simulink model "ADCS_r2017b"  (R2018a)
settings: Solver=FixedStepAuto  StartTime=0.0  StopTime=end_time  FixedStep=delta_t  RelTol=1e-3
undefined symbols (not defined in the file or in its folder): delta_t, SC, SS
libraries: sharedutil x5, vrlib x2
(part 1 of 3)
settings Model: Creator=azufall  LastModifiedBy=Hridu
settings DebuggingCC: AlgebraicLoopMsg=none

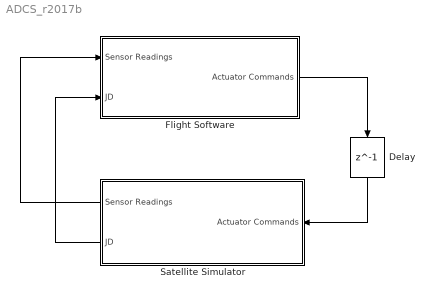
== system ADCS_r2017b ==
  Delay : Delay  DelayLength=1  InitialCondition=0
  Flight Software : Subsystem
  Satellite Simulator : Subsystem
  wires:
  Flight Software/1(Actuator Commands) -> Delay/1
  Satellite Simulator/2(JD) -> Flight Software/2(JD)
  Satellite Simulator/1(Sensor Readings) -> Flight Software/1(Sensor Readings)
  Delay/1 -> Satellite Simulator/1(Actuator Commands)

== system ADCS_r2017b/Flight Software ==
  Sensor Readings : Inport
  JD : Inport  Port=2
  Bus Selector : BusSelector  OutputSignals=gyro meas,sun meas,star meas
  Resolution Error : Rounding
  Subsystems : Subsystem
  Thrust command : Gain  Gain=SC.RCS.num_bits
  Thrust command1 : Gain  Gain=1/SC.RCS.num_bits
  Actuator Commands : Outport
  wires:
  Subsystems/1(RCS Command) -> Thrust command/1
  Sensor Readings/1 -> Bus Selector/1
  Bus Selector/1 -> Subsystems/1(Gyro)  "<gyro meas>"
  Bus Selector/3 -> Subsystems/3(Star Tracker)  "<star meas>"
  JD/1 -> Subsystems/4(JD)
  Thrust command/1 -> Resolution Error/1
  Resolution Error/1 -> Thrust command1/1
  Bus Selector/2 -> Subsystems/2(Sun Sensor)  "<sun meas>"
  Thrust command1/1 -> Actuator Commands/1

== system ADCS_r2017b/Satellite Simulator ==
  Actuator Commands : Inport
  Actuators : Subsystem
  Constant : Constant  Value=0
  Constant1 : Constant  Value=[0;0;0]
  Constant2 : Constant  Value=[0;0;0]
  Delay : Delay  DelayLength=1  InitialConditionSource=Input port  InitialCondition=0
      settings: InputPortMap=u0,p4
  Delay1 : Delay  DelayLength=1  InitialConditionSource=Input port  InitialCondition=0
      settings: InputPortMap=u0,p4
  Environment : Subsystem
  External Forces and Torques : Subsystem
  Kinematics : Subsystem
  Sensors : Subsystem
  Sum : Sum  Inputs=++|
  Sum1 : Sum  Inputs=++|
  Time Model : Subsystem
  Sensor Readings : Outport
  JD : Outport  Port=2  PortDimensions=1
  wires:
  Kinematics/3(Omega) -> Sensors/3(w_body2eci)
  Sensors/1(Sensor Readings) -> Sensor Readings/1
  Time Model/1(JD) -> External Forces and Torques/8(JD), Kinematics/3(JD), Environment/1(JD), JD/1
  Environment/1(sun_eci) -> Sensors/2(Sun info), External Forces and Torques/4(sun_eci)
  Environment/2(moon_eci) -> External Forces and Torques/5(moon_eci)
  Environment/3(Mag) -> External Forces and Torques/6(Mag)
  External Forces and Torques/1(a_eci) -> Sum/2
  External Forces and Torques/2(tor_body) -> Sum1/2
  Kinematics/2(v_eci) -> External Forces and Torques/2(Velocity)
  Kinematics/4(Coordinate Transforms) -> Environment/3(Coordinate Transforms), Sensors/4(Coordinate Transforms), Actuators/3(Coordinate Transforms), External Forces and Torques/3(Coordinate Transforms)
  Actuators/1(a_eci) -> Sum/1
  Actuators/2(torque_body) -> Sum1/1
  Kinematics/1(r_eci) -> Sensors/1(Position), Environment/2(r_eci), External Forces and Torques/1(Position)
  Environment/4(Eclipse) -> Sensors/6(eclipse), External Forces and Torques/7(Eclipse)
  Kinematics/5(q) -> Sensors/5(q_eci2body)
  Actuator Commands/1 -> Actuators/1(RCS Command)
  Constant/1 -> Actuators/2(Other Actuator?)
  Sum1/1 -> Delay/1
  Sum/1 -> Delay1/1
  Delay1/1 -> Kinematics/1(a_eci)
  Constant1/1 -> Delay1/2
  Constant2/1 -> Delay/2
  Delay/1 -> Kinematics/2(Torque_body)

== system ADCS_r2017b/Flight Software/Subsystems ==
  Gyro : Inport
  Sun Sensor : Inport  Port=2
  Star Tracker : Inport  Port=3
  JD : Inport  Port=4
  Mode Selection : Subsystem
  RCS Controller : Subsystem
  Sensor Processing : Subsystem
  To Workspace : ToWorkspace  VariableName=mode_out  SampleTime=-1
  RCS Command : Outport
  wires:
  Gyro/1 -> Sensor Processing/1(Gyro_raw)
  Sun Sensor/1 -> Sensor Processing/2(Sun_raw)
  Star Tracker/1 -> Sensor Processing/3(Star_raw)
  Sensor Processing/1(Gyro_filtered) -> RCS Controller/2(Gyro), Mode Selection/1(Gyro)
  Sensor Processing/4(Eclipse) -> RCS Controller/7(eclipse), Mode Selection/2(Eclipse)
  JD/1 -> RCS Controller/6(JD), Mode Selection/3(Time)
  RCS Controller/1(RCS_Command) -> RCS Command/1
  Mode Selection/2(S/C Mode) -> To Workspace/1, RCS Controller/1(Mode)
  Mode Selection/1(Controller Gains) -> RCS Controller/5(Gains)
  Sensor Processing/3(Star_filtered) -> RCS Controller/4(Star)
  Sensor Processing/2(Sun_filtered) -> RCS Controller/3(Sun)

== system ADCS_r2017b/Satellite Simulator/Actuators ==
  RCS Command : Inport
  Other Actuator? : Inport  Port=2
  Coordinate Transforms : Inport  Port=3
  Bus Selector : BusSelector  OutputSignals=R_eci2body
  Constant : Constant  Value=SC.RCS.moment_arms
  Constant1 : Constant  Value=SC.RCS.max_thrust
  Constant2 : Constant  Value=SC.RCS.dir
  Constant3 : Constant  Value=SC.RCS.noise
  Constant4 : Constant  Value=SC.RCS.bias
  Gain : Gain  Gain=1/SC.mass_properties.mass
  Math Function : Math  Operator=transpose  SaturateOnIntegerOverflow=on
  Matrix Multiply : Product  Multiplication=Matrix(*)
  RCS Model : MATLAB Function  TreatAsAtomicUnit=on
  Terminator : Terminator
  To Workspace : ToWorkspace  VariableName=act_tor_body  SampleTime=-1
  To Workspace1 : ToWorkspace  VariableName=RCS_cmds  SampleTime=-1
  a_eci : Outport
  torque_body : Outport  Port=2
  wires:
  RCS Command/1 -> To Workspace1/1, RCS Model/1(command)
  RCS Model/2(torque_body) -> To Workspace/1, torque_body/1
  Other Actuator?/1 -> Terminator/1
  Coordinate Transforms/1 -> Bus Selector/1
  Bus Selector/1 -> Math Function/1  "<R_eci2body>"
  RCS Model/1(force_body) -> Matrix Multiply/2
  Math Function/1 -> Matrix Multiply/1  "R_body2eci"
  Constant/1 -> RCS Model/2(moment_arm)
  Constant1/1 -> RCS Model/4(max_thrust)
  Constant2/1 -> RCS Model/3(norm_dir)
  Gain/1 -> a_eci/1
  Matrix Multiply/1 -> Gain/1
  Constant3/1 -> RCS Model/5(noise)
  Constant4/1 -> RCS Model/6(bias)

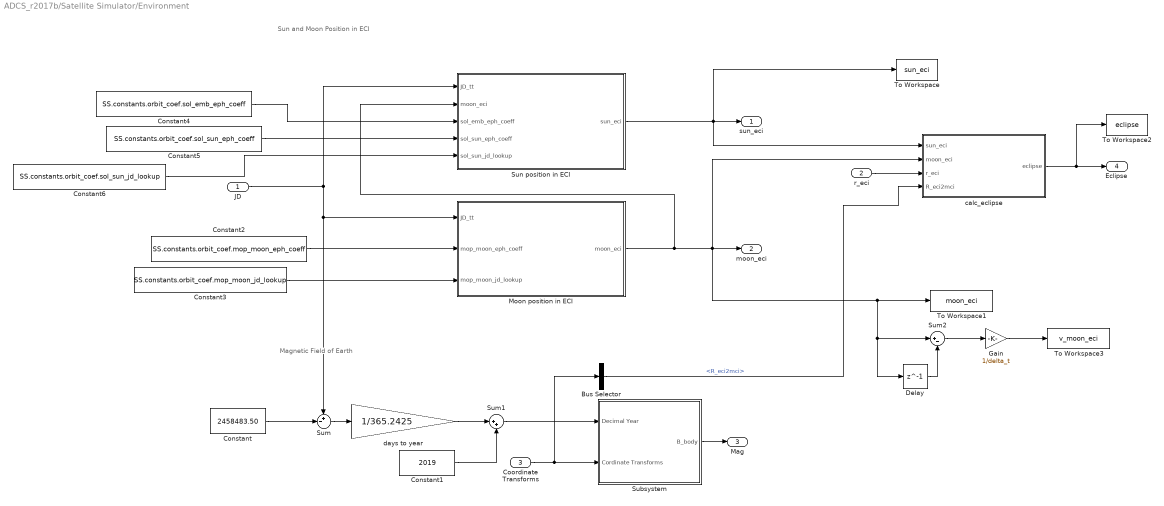
== system ADCS_r2017b/Satellite Simulator/Environment ==
  note: Sun and Moon Position in ECI
  note: Magnetic Field of Earth
  JD : Inport
  r_eci : Inport  Port=2
  Coordinate Transforms : Inport  Port=3
  Bus Selector : BusSelector  OutputSignals=R_eci2mci
  Constant : Constant  Value=2458483.50
  Constant1 : Constant  Value=2019
  Constant2 : Constant  Value=SS.constants.orbit_coef.mop_moon_eph_coeff
  Constant3 : Constant  Value=SS.constants.orbit_coef.mop_moon_jd_lookup
  Constant4 : Constant  Value=SS.constants.orbit_coef.sol_emb_eph_coeff
  Constant5 : Constant  Value=SS.constants.orbit_coef.sol_sun_eph_coeff
  Constant6 : Constant  Value=SS.constants.orbit_coef.sol_sun_jd_lookup
  Delay : Delay  DelayLength=1  InitialCondition=0
  Gain : Gain  Gain=1/delta_t
  Moon position in ECI : MATLAB Function  TreatAsAtomicUnit=on
  Subsystem : Subsystem
  Sum : Sum  Inputs=+-|
  Sum1 : Sum  Inputs=|++
  Sum2 : Sum  Inputs=|+-
  Sun position in ECI : MATLAB Function  TreatAsAtomicUnit=on
  To Workspace : ToWorkspace  VariableName=sun_eci  SampleTime=-1
  To Workspace1 : ToWorkspace  VariableName=moon_eci  SampleTime=-1
  To Workspace2 : ToWorkspace  VariableName=eclipse  SampleTime=-1
  To Workspace3 : ToWorkspace  VariableName=v_moon_eci  SampleTime=-1
  calc_eclipse : MATLAB Function  TreatAsAtomicUnit=on
  days to year : Gain  Gain=1/365.2425
  sun_eci : Outport
  moon_eci : Outport  Port=2
  Mag : Outport  Port=3
  Eclipse : Outport  Port=4
  wires:
  Moon position in ECI/1(moon_eci) -> Sun position in ECI/2(moon_eci), calc_eclipse/2(moon_eci), moon_eci/1, Delay/1, Sum2/1, To Workspace1/1
  Subsystem/1(B_body) -> Mag/1
  calc_eclipse/1(eclipse) -> To Workspace2/1, Eclipse/1
  JD/1 -> Sum/1, Moon position in ECI/1(JD_tt), Sun position in ECI/1(JD_tt)
  Sun position in ECI/1(sun_eci) -> sun_eci/1, To Workspace/1, calc_eclipse/1(sun_eci)
  r_eci/1 -> calc_eclipse/3(r_eci)
  Sum/1 -> days to year/1
  Constant/1 -> Sum/2
  days to year/1 -> Sum1/1
  Sum1/1 -> Subsystem/1(Decimal Year)
  Constant1/1 -> Sum1/2
  Coordinate Transforms/1 -> Bus Selector/1, Subsystem/2(Cordinate Transforms)
  Constant2/1 -> Moon position in ECI/2(mop_moon_eph_coeff)
  Constant3/1 -> Moon position in ECI/3(mop_moon_jd_lookup)
  Constant4/1 -> Sun position in ECI/3(sol_emb_eph_coeff)
  Constant5/1 -> Sun position in ECI/4(sol_sun_eph_coeff)
  Constant6/1 -> Sun position in ECI/5(sol_sun_jd_lookup)
  Bus Selector/1 -> calc_eclipse/4(R_eci2mci)  "<R_eci2mci>"
  Delay/1 -> Sum2/2
  Sum2/1 -> Gain/1
  Gain/1 -> To Workspace3/1

== system ADCS_r2017b/Satellite Simulator/External Forces and Torques ==
  Position : Inport
  Velocity : Inport  Port=2
  Coordinate Transforms : Inport  Port=3
  sun_eci : Inport  Port=4
  moon_eci : Inport  Port=5
  Mag : Inport  Port=6
  Eclipse : Inport  Port=7
  JD : Inport  Port=8
  External Forces : Subsystem
  External Torques : Subsystem
  a_eci : Outport
  tor_body : Outport  Port=2
  wires:
  Position/1 -> External Forces/1(r_eci), External Torques/3(r_eci)
  moon_eci/1 -> External Forces/5(moon eci)
  sun_eci/1 -> External Forces/4(Sun eci)
  Velocity/1 -> External Forces/2(Velocity)
  Coordinate Transforms/1 -> External Torques/5(Coordinate Transforms), External Forces/3(Coordinate Transforms)
  External Forces/1(a_eci) -> a_eci/1
  External Torques/1(Torques) -> tor_body/1
  Eclipse/1 -> External Forces/6(Eclipse)
  Mag/1 -> External Torques/4(Mag)
  External Forces/2(Aero_body) -> External Torques/1(Force_aero_body)
  External Forces/3(SRP_body) -> External Torques/2(Force_SRP_body)
  JD/1 -> External Forces/7(JD)

== system ADCS_r2017b/Satellite Simulator/Kinematics ==
  a_eci : Inport
  Torque_body : Inport  Port=2
  JD : Inport  Port=3  PortDimensions=1
  Backup Rotation Kinematics : Subsystem
  Calc Coordinate Transforms : Subsystem
  Position Kinematics : Subsystem
  Rotation Kinematics : Subsystem
  To Workspace : ToWorkspace  VariableName=q_out  SampleTime=-1
  To Workspace1 : ToWorkspace  VariableName=omega_out  SampleTime=-1
  To Workspace2 : ToWorkspace  VariableName=e_out  SampleTime=-1
  To Workspace3 : ToWorkspace  VariableName=omega_euler_out  SampleTime=-1
  r_eci : Outport
  v_eci : Outport  Port=2
  Omega : Outport  Port=3
  Coordinate Transforms : Outport  Port=4
  q : Outport  Port=5
  wires:
  a_eci/1 -> Position Kinematics/1(a_eci)
  Torque_body/1 -> Backup Rotation Kinematics/1(torque_body), Rotation Kinematics/1(torque_body)
  Rotation Kinematics/2(w_body_eci) -> To Workspace1/1, Omega/1
  Calc Coordinate Transforms/1(Coordinate Transforms) -> Coordinate Transforms/1
  Backup Rotation Kinematics/1(euler_angles) -> To Workspace2/1
  Backup Rotation Kinematics/2(w_body_eci) -> To Workspace3/1
  Position Kinematics/1(r_eci) -> Calc Coordinate Transforms/1(r_eci), r_eci/1
  Position Kinematics/2(v_eci) -> Calc Coordinate Transforms/2(Velocity), v_eci/1
  Rotation Kinematics/1(q) -> To Workspace/1, Calc Coordinate Transforms/4(Attitude), q/1
  JD/1 -> Calc Coordinate Transforms/3(JD)

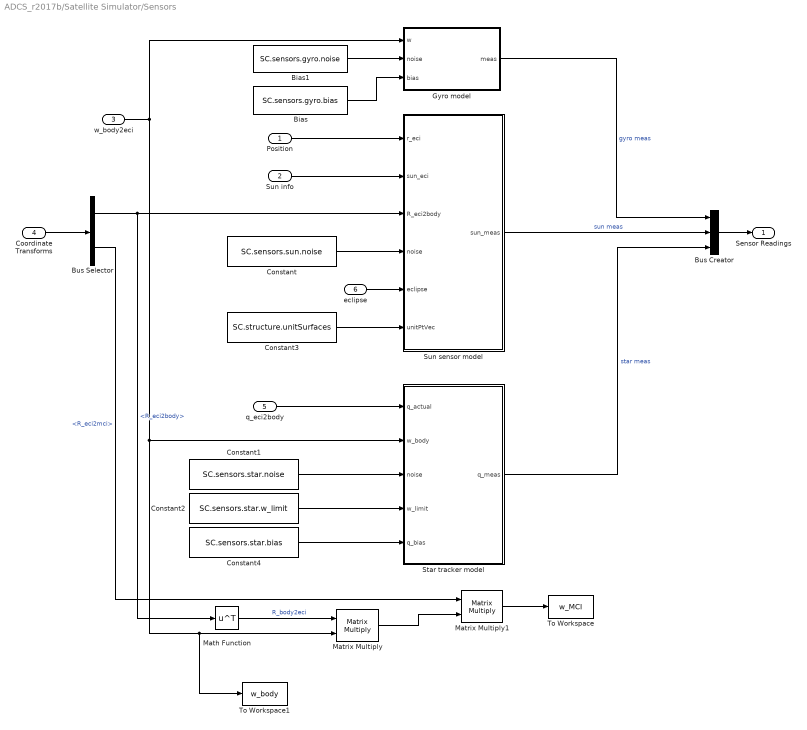
== system ADCS_r2017b/Satellite Simulator/Sensors ==
  Position : Inport
  Sun info : Inport  Port=2
  w_body2eci : Inport  Port=3
  Coordinate Transforms : Inport  Port=4
  q_eci2body : Inport  Port=5
  eclipse : Inport  Port=6
  Bias : Constant  Value=SC.sensors.gyro.bias
  Bias1 : Constant  Value=SC.sensors.gyro.noise
  Bus Creator : BusCreator  Inputs=3
  Bus Selector : BusSelector  OutputSignals=R_eci2body,R_eci2mci
  Constant : Constant  Value=SC.sensors.sun.noise
  Constant1 : Constant  Value=SC.sensors.star.noise
  Constant2 : Constant  Value=SC.sensors.star.w_limit
  Constant3 : Constant  Value=SC.structure.unitSurfaces
  Constant4 : Constant  Value=SC.sensors.star.bias
  Gyro model : MATLAB Function  TreatAsAtomicUnit=on
  Math Function : Math  Operator=transpose  SaturateOnIntegerOverflow=on
  Matrix Multiply : Product  Multiplication=Matrix(*)
  Matrix Multiply1 : Product  Multiplication=Matrix(*)
  Star tracker model : MATLAB Function  TreatAsAtomicUnit=on
  Sun sensor model : MATLAB Function  TreatAsAtomicUnit=on
  To Workspace : ToWorkspace  VariableName=w_MCI  SampleTime=-1
  To Workspace1 : ToWorkspace  VariableName=w_body  SampleTime=-1
  Sensor Readings : Outport
  wires:
  Bus Creator/1 -> Sensor Readings/1
  Star tracker model/1(q_meas) -> Bus Creator/3  "star meas"
  Sun info/1 -> Sun sensor model/2(sun_eci)
  Position/1 -> Sun sensor model/1(r_eci)
  Constant/1 -> Sun sensor model/4(noise)
  Sun sensor model/1(sun_meas) -> Bus Creator/2  "sun meas"
  w_body2eci/1 -> Gyro model/1(w), To Workspace1/1, Matrix Multiply/2, Star tracker model/2(w_body)
  Gyro model/1(meas) -> Bus Creator/1  "gyro meas"
  Constant1/1 -> Star tracker model/3(noise)
  Constant2/1 -> Star tracker model/4(w_limit)
  eclipse/1 -> Sun sensor model/5(eclipse)
  Coordinate Transforms/1 -> Bus Selector/1
  Bus Selector/1 -> Math Function/1, Sun sensor model/3(R_eci2body)  "<R_eci2body>"
  Constant3/1 -> Sun sensor model/6(unitPtVec)
  q_eci2body/1 -> Star tracker model/1(q_actual)
  Math Function/1 -> Matrix Multiply/1  "R_body2eci"
  Matrix Multiply/1 -> Matrix Multiply1/2
  Bus Selector/2 -> Matrix Multiply1/1  "<R_eci2mci>"
  Matrix Multiply1/1 -> To Workspace/1
  Constant4/1 -> Star tracker model/5(q_bias)
  Bias1/1 -> Gyro model/2(noise)
  Bias/1 -> Gyro model/3(bias)

== system ADCS_r2017b/Satellite Simulator/Time Model ==
  Constant : Constant  Value=SC.initial_state.date  VectorParams1D=off
  Constant1 : Constant  Value=delta_t
  Date2JD : MATLAB Function  TreatAsAtomicUnit=on
  Delay : Delay  DelayLength=1  InitialConditionSource=Input port  InitialCondition=0
      settings: InputPortMap=u0,p4
  Sum : Sum  Inputs=|++  InputSameDT=on
  To Workspace : ToWorkspace  VariableName=JD  SampleTime=-1
  days per second : Gain  Gain=1/(24*60*60)
  JD : Outport
  wires:
  Sum/1 -> To Workspace/1, JD/1, Delay/1
  Constant1/1 -> days per second/1
  Delay/1 -> Sum/1
  Constant/1 -> Date2JD/1(date)
  Date2JD/1(JD) -> Delay/2
  days per second/1 -> Sum/2

== system ADCS_r2017b/Flight Software/Subsystems/Mode Selection ==
  Gyro : Inport
  Eclipse : Inport  Port=2
  Time : Inport  Port=3
  3_axis_gains : Constant  Value=SC.ax3.gains
  3_axis_gains1 : Constant  Value=SC.spin.gains
  3_axis_gains2 : Constant  Value=SC.ax3.time_constant
  3_axis_gains3 : Constant  Value=SC.spin.time_constant
  3_axis_gains4 : Constant  Value=SC.spin_up.time_constant
  3_axis_gains5 : Constant  Value=SC.spin_up.gains
  Bus Creator : BusCreator  Inputs=2
  MATLAB Function : MATLAB Function  TreatAsAtomicUnit=on
  Controller Gains : Outport
  S/C Mode : Outport  Port=2
  wires:
  Time/1 -> MATLAB Function/3(JD)
  Gyro/1 -> MATLAB Function/1(gyro)
  Eclipse/1 -> MATLAB Function/2(eclipse)
  MATLAB Function/3(mode) -> S/C Mode/1
  3_axis_gains/1 -> MATLAB Function/4(ax3_gains)
  3_axis_gains2/1 -> MATLAB Function/5(ax3_TC)
  3_axis_gains1/1 -> MATLAB Function/6(spin_gains)
  3_axis_gains3/1 -> MATLAB Function/7(spin_TC)
  3_axis_gains5/1 -> MATLAB Function/8(spin_up_gains)
  3_axis_gains4/1 -> MATLAB Function/9(spin_up_TC)
  Bus Creator/1 -> Controller Gains/1
  MATLAB Function/2(Kd) -> Bus Creator/2
  MATLAB Function/1(Kp) -> Bus Creator/1

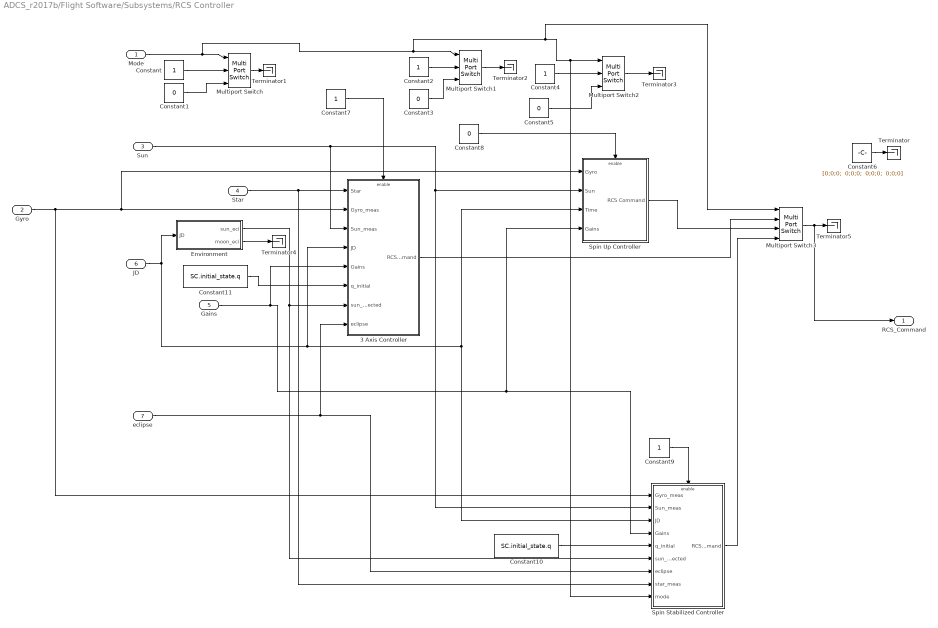
== system ADCS_r2017b/Flight Software/Subsystems/RCS Controller ==
  Mode : Inport
  Gyro : Inport  Port=2
  Sun : Inport  Port=3
  Star : Inport  Port=4
  Gains : Inport  Port=5
  JD : Inport  Port=6
  eclipse : Inport  Port=7
  3 Axis Controller : Subsystem  TreatAsAtomicUnit=on
  Constant{,2,4,7,9} (5 alike) : Constant
  Constant{1,3,5,8} (4 alike) : Constant  Value=0
  Constant10 : Constant  Value=SC.initial_state.q
  Constant11 : Constant  Value=SC.initial_state.q
  Constant6 : Constant  Value="[0;0;0;  0;0;0;  0;0;0;  0;0;0]"
  Environment : Subsystem
  Multiport Switch : MultiPortSwitch  Inputs=2
  Multiport Switch1 : MultiPortSwitch  Inputs=2
  Multiport Switch2 : MultiPortSwitch  Inputs=2
  Multiport Switch3 : MultiPortSwitch  DiagnosticForDefault=None
  Spin Stabilized Controller : Subsystem  TreatAsAtomicUnit=on
  Spin Up Controller : Subsystem  TreatAsAtomicUnit=on
  Terminator{,1..5} (6 alike) : Terminator
  RCS_Command : Outport
  wires:
  Mode/1 -> Multiport Switch3/1, Spin Stabilized Controller/9(mode), Multiport Switch2/1, Multiport Switch1/1, Multiport Switch/1
  Sun/1 -> 3 Axis Controller/3(Sun_meas), Spin Stabilized Controller/2(Sun_meas), Spin Up Controller/2(Sun)
  JD/1 -> Environment/1(JD), 3 Axis Controller/4(JD), Spin Up Controller/3(Time), Spin Stabilized Controller/3(JD)
  Gains/1 -> 3 Axis Controller/5(Gains), Spin Stabilized Controller/4(Gains), Spin Up Controller/4(Gains)
  Spin Up Controller/1(RCS Command) -> Multiport Switch3/3
  Spin Stabilized Controller/1(RCS Command) -> Multiport Switch3/4
  Constant/1 -> Multiport Switch/2
  Constant1/1 -> Multiport Switch/3
  Constant2/1 -> Multiport Switch1/2
  Constant3/1 -> Multiport Switch1/3
  Constant4/1 -> Multiport Switch2/2
  Constant5/1 -> Multiport Switch2/3
  Constant7/1 -> 3 Axis Controller/Enable
  Constant8/1 -> Spin Up Controller/Enable
  Constant9/1 -> Spin Stabilized Controller/Enable
  Multiport Switch/1 -> Terminator1/1
  Multiport Switch1/1 -> Terminator2/1
  Multiport Switch2/1 -> Terminator3/1
  Environment/1(sun_eci) -> Spin Stabilized Controller/6(sun_expected), 3 Axis Controller/7(sun_expected)
  Environment/2(moon_eci) -> Terminator4/1
  Constant10/1 -> Spin Stabilized Controller/5(q_initial)
  eclipse/1 -> 3 Axis Controller/8(eclipse), Spin Stabilized Controller/7(eclipse)
  Constant11/1 -> 3 Axis Controller/6(q_initial)
  Gyro/1 -> Spin Stabilized Controller/1(Gyro_meas), Spin Up Controller/1(Gyro), 3 Axis Controller/2(Gyro_meas)
  Constant6/1 -> Terminator/1
  Multiport Switch3/1 -> RCS_Command/1, Terminator5/1
  3 Axis Controller/1(RCS Command) -> Multiport Switch3/2
  Star/1 -> Spin Stabilized Controller/8(star_meas), 3 Axis Controller/1(Star)

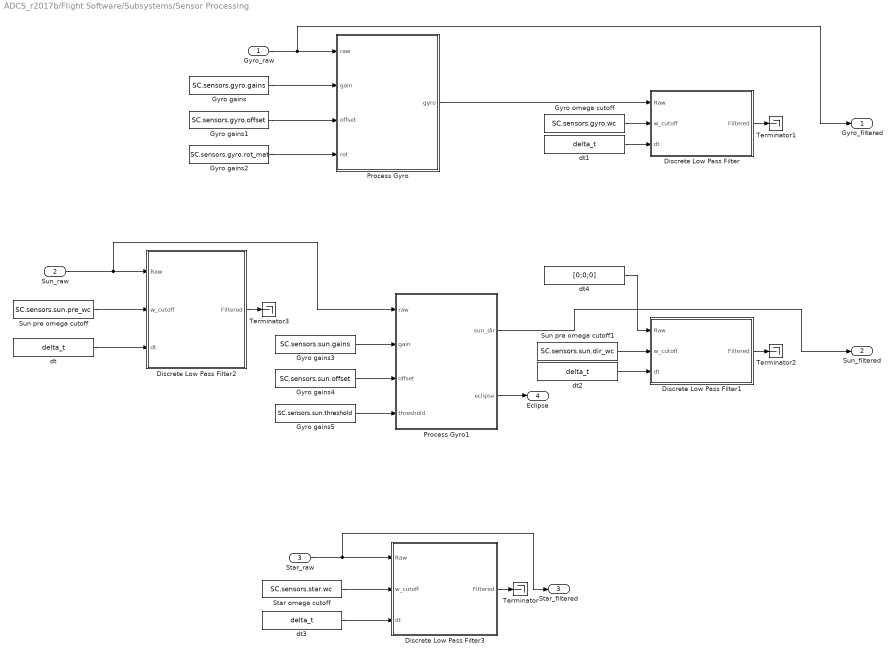
== system ADCS_r2017b/Flight Software/Subsystems/Sensor Processing ==
  Gyro_raw : Inport
  Sun_raw : Inport  Port=2
  Star_raw : Inport  Port=3
  Discrete Low Pass Filter : Subsystem
  Discrete Low Pass Filter1 : Subsystem
  Discrete Low Pass Filter2 : Subsystem
  Discrete Low Pass Filter3 : Subsystem
  Gyro gains : Constant  Value=SC.sensors.gyro.gains
  Gyro gains1 : Constant  Value=SC.sensors.gyro.offset
  Gyro gains2 : Constant  Value=SC.sensors.gyro.rot_mat
  Gyro gains3 : Constant  Value=SC.sensors.sun.gains
  Gyro gains4 : Constant  Value=SC.sensors.sun.offset
  Gyro gains5 : Constant  Value=SC.sensors.sun.threshold
  Gyro omega cutoff : Constant  Value=SC.sensors.gyro.wc
  Process Gyro : MATLAB Function  TreatAsAtomicUnit=on
  Process Gyro1 : MATLAB Function  TreatAsAtomicUnit=on
  Star omega cutoff : Constant  Value=SC.sensors.star.wc
  Sun pre omega cutoff : Constant  Value=SC.sensors.sun.pre_wc
  Sun pre omega cutoff1 : Constant  Value=SC.sensors.sun.dir_wc
  Terminator{,1..3} (4 alike) : Terminator
  dt{,1..3} (4 alike) : Constant  Value=delta_t
  dt4 : Constant  Value=[0;0;0]
  Gyro_filtered : Outport
  Sun_filtered : Outport  Port=2
  Star_filtered : Outport  Port=3
  Eclipse : Outport  Port=4
  wires:
  Gyro_raw/1 -> Gyro_filtered/1, Process Gyro/1(raw)
  Gyro gains/1 -> Process Gyro/2(gain)
  Gyro gains1/1 -> Process Gyro/3(offset)
  Gyro gains2/1 -> Process Gyro/4(rot)
  Process Gyro/1(gyro) -> Discrete Low Pass Filter/1(Raw)
  Gyro omega cutoff/1 -> Discrete Low Pass Filter/2(w_cutoff)
  dt1/1 -> Discrete Low Pass Filter/3(dt)
  Sun_raw/1 -> Process Gyro1/1(raw), Discrete Low Pass Filter2/1(Raw)
  Process Gyro1/2(eclipse) -> Eclipse/1
  Sun pre omega cutoff/1 -> Discrete Low Pass Filter2/2(w_cutoff)
  dt/1 -> Discrete Low Pass Filter2/3(dt)
  Gyro gains3/1 -> Process Gyro1/2(gain)
  Gyro gains4/1 -> Process Gyro1/3(offset)
  Gyro gains5/1 -> Process Gyro1/4(threshold)
  Sun pre omega cutoff1/1 -> Discrete Low Pass Filter1/2(w_cutoff)
  dt2/1 -> Discrete Low Pass Filter1/3(dt)
  Star_raw/1 -> Star_filtered/1, Discrete Low Pass Filter3/1(Raw)
  Star omega cutoff/1 -> Discrete Low Pass Filter3/2(w_cutoff)
  dt3/1 -> Discrete Low Pass Filter3/3(dt)
  Discrete Low Pass Filter3/1(Filtered) -> Terminator/1
  Discrete Low Pass Filter/1(Filtered) -> Terminator1/1
  Discrete Low Pass Filter1/1(Filtered) -> Terminator2/1
  Process Gyro1/1(sun_dir) -> Sun_filtered/1
  Discrete Low Pass Filter2/1(Filtered) -> Terminator3/1
  dt4/1 -> Discrete Low Pass Filter1/1(Raw)

== system ADCS_r2017b/Satellite Simulator/Environment/Subsystem ==
  Decimal Year : Inport
  Cordinate Transforms : Inport  Port=2
  Bus Selector : BusSelector  OutputSignals=R_eci2ecef,R_eci2body,geod,R_ecef2ned
  Bus Selector1 : BusSelector  OutputSignals=phi,lambda,h
  Constant : Constant  Value=SS.constants.igrf.yearLastEpoch
  Constant1 : Constant  Value=SS.constants.igrf.lastgh
  Constant2 : Constant  Value=SS.constants.igrf.ghslope
  MATLAB Function : MATLAB Function  TreatAsAtomicUnit=on
  Math Function : Math  Operator=transpose  SaturateOnIntegerOverflow=on
  Math Function1 : Math  Operator=transpose  SaturateOnIntegerOverflow=on
  Matrix Multiply : Product  Multiplication=Matrix(*)
  Matrix Multiply1 : Product  Multiplication=Matrix(*)
  Matrix Multiply2 : Product  Multiplication=Matrix(*)
  B_body : Outport
  wires:
  Cordinate Transforms/1 -> Bus Selector/1
  Bus Selector/4 -> Math Function/1  "<R_ecef2ned>"
  MATLAB Function/1(B_ned) -> Matrix Multiply/2
  Math Function/1 -> Matrix Multiply/1
  Bus Selector/3 -> Bus Selector1/1  "<geod>"
  Bus Selector/2 -> Matrix Multiply2/1  "<R_eci2body>"
  Bus Selector/1 -> Math Function1/1  "<R_eci2ecef>"
  Matrix Multiply/1 -> Matrix Multiply1/2  "B_ecef"
  Matrix Multiply1/1 -> Matrix Multiply2/2  "B_eci"
  Matrix Multiply2/1 -> B_body/1
  Math Function1/1 -> Matrix Multiply1/1
  Decimal Year/1 -> MATLAB Function/1(decYear)
  Bus Selector1/3 -> MATLAB Function/7(altitude)  "<h>"
  Bus Selector1/1 -> MATLAB Function/5(latitude)  "<phi>"
  Bus Selector1/2 -> MATLAB Function/6(longitude)  "<lambda>"
  Constant/1 -> MATLAB Function/2(yearLastEpoch)
  Constant1/1 -> MATLAB Function/3(lastgh)
  Constant2/1 -> MATLAB Function/4(ghslope)

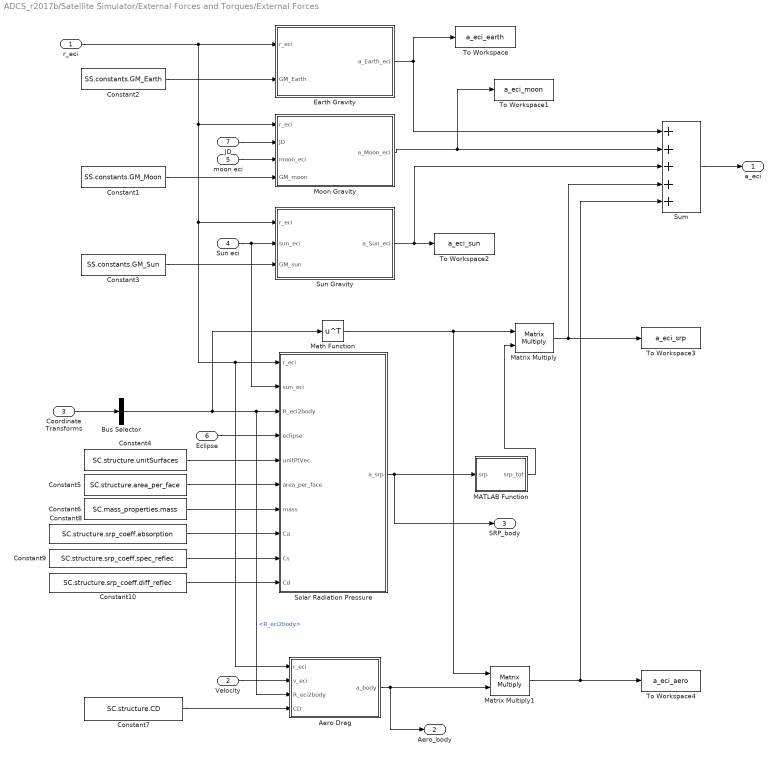
== system ADCS_r2017b/Satellite Simulator/External Forces and Torques/External Forces ==
  r_eci : Inport
  Velocity : Inport  Port=2
  Coordinate Transforms : Inport  Port=3
  Sun eci : Inport  Port=4
  moon eci : Inport  Port=5
  Eclipse : Inport  Port=6
  JD : Inport  Port=7  PortDimensions=1
  Aero Drag : MATLAB Function  TreatAsAtomicUnit=on
  Bus Selector : BusSelector  OutputSignals=R_eci2body
  Constant1 : Constant  Value=SS.constants.GM_Moon
  Constant10 : Constant  Value=SC.structure.srp_coeff.diff_reflec
  Constant2 : Constant  Value=SS.constants.GM_Earth
  Constant3 : Constant  Value=SS.constants.GM_Sun
  Constant4 : Constant  Value=SC.structure.unitSurfaces
  Constant5 : Constant  Value=SC.structure.area_per_face
  Constant6 : Constant  Value=SC.mass_properties.mass
  Constant7 : Constant  Value=SC.structure.CD
  Constant8 : Constant  Value=SC.structure.srp_coeff.absorption
  Constant9 : Constant  Value=SC.structure.srp_coeff.spec_reflec
  Earth Gravity : MATLAB Function  TreatAsAtomicUnit=on
  MATLAB Function : MATLAB Function  TreatAsAtomicUnit=on
  Math Function : Math  Operator=transpose  SaturateOnIntegerOverflow=on
  Matrix Multiply : Product  Multiplication=Matrix(*)
  Matrix Multiply1 : Product  Multiplication=Matrix(*)
  Moon Gravity : MATLAB Function  TreatAsAtomicUnit=on
  Solar Radiation Pressure : MATLAB Function  TreatAsAtomicUnit=on
  Sum : Sum  Inputs=+++++
  Sun Gravity : MATLAB Function  TreatAsAtomicUnit=on
  To Workspace : ToWorkspace  VariableName=a_eci_earth  SampleTime=-1
  To Workspace1 : ToWorkspace  VariableName=a_eci_moon  SampleTime=-1
  To Workspace2 : ToWorkspace  VariableName=a_eci_sun  SampleTime=-1
  To Workspace3 : ToWorkspace  VariableName=a_eci_srp  SampleTime=-1
  To Workspace4 : ToWorkspace  VariableName=a_eci_aero  SampleTime=-1
  a_eci : Outport
  Aero_body : Outport  Port=2
  SRP_body : Outport  Port=3
  wires:
  Sun eci/1 -> Sun Gravity/2(sun_eci), Solar Radiation Pressure/2(sun_eci)
  Solar Radiation Pressure/1(a_srp) -> SRP_body/1, MATLAB Function/1(srp)
  Sum/1 -> a_eci/1
  Earth Gravity/1(a_Earth_eci) -> Sum/1, To Workspace/1
  Sun Gravity/1(a_Sun_eci) -> To Workspace2/1, Sum/3
  Velocity/1 -> Aero Drag/2(v_eci)
  Coordinate Transforms/1 -> Bus Selector/1
  Moon Gravity/1(a_Moon_eci) -> To Workspace1/1, Sum/2
  r_eci/1 -> Aero Drag/1(r_eci), Solar Radiation Pressure/1(r_eci), Sun Gravity/1(r_eci), Moon Gravity/1(r_eci), Earth Gravity/1(r_eci)
  Bus Selector/1 -> Math Function/1, Aero Drag/3(R_eci2body), Solar Radiation Pressure/3(R_eci2body)  "<R_eci2body>"
  Constant2/1 -> Earth Gravity/2(GM_Earth)
  Constant3/1 -> Sun Gravity/3(GM_sun)
  Eclipse/1 -> Solar Radiation Pressure/4(eclipse)
  Constant4/1 -> Solar Radiation Pressure/5(unitPtVec)
  Constant5/1 -> Solar Radiation Pressure/6(area_per_face)
  Constant6/1 -> Solar Radiation Pressure/7(mass)
  Constant7/1 -> Aero Drag/4(CD)
  Matrix Multiply/1 -> To Workspace3/1, Sum/4
  Math Function/1 -> Matrix Multiply1/1, Matrix Multiply/1
  Aero Drag/1(a_body) -> Aero_body/1, Matrix Multiply1/2
  Matrix Multiply1/1 -> To Workspace4/1, Sum/5
  Constant8/1 -> Solar Radiation Pressure/8(Ca)
  Constant9/1 -> Solar Radiation Pressure/9(Cs)
  Constant10/1 -> Solar Radiation Pressure/10(Cd)
  MATLAB Function/1(srp_tot) -> Matrix Multiply/2
  JD/1 -> Moon Gravity/2(JD)
  Constant1/1 -> Moon Gravity/4(GM_moon)
  moon eci/1 -> Moon Gravity/3(moon_eci)

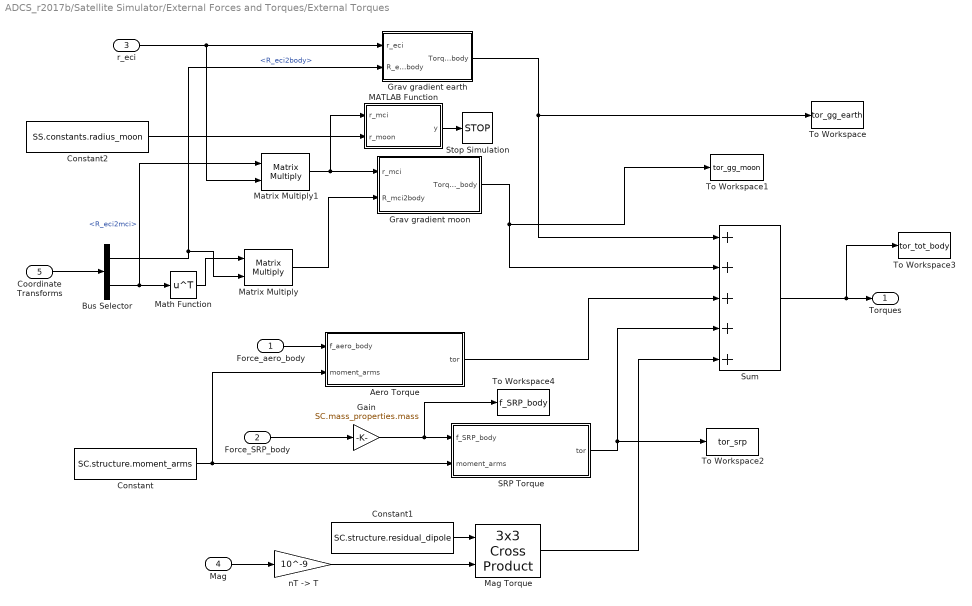
== system ADCS_r2017b/Satellite Simulator/External Forces and Torques/External Torques ==
  Force_aero_body : Inport
  Force_SRP_body : Inport  Port=2
  r_eci : Inport  Port=3
  Mag : Inport  Port=4
  Coordinate Transforms : Inport  Port=5
  Aero Torque : MATLAB Function  TreatAsAtomicUnit=on
  Bus Selector : BusSelector  OutputSignals=R_eci2body,R_eci2mci
  Constant : Constant  Value=SC.structure.moment_arms
  Constant1 : Constant  Value=SC.structure.residual_dipole
  Constant2 : Constant  Value=SS.constants.radius_moon
  Gain : Gain  Gain=SC.mass_properties.mass
  Grav gradient earth : Subsystem
  Grav gradient moon : Subsystem
  MATLAB Function : MATLAB Function  TreatAsAtomicUnit=on
  Mag Torque : sharedutil/3x3 Cross Product  aMode=aMode
      settings: SourceProductBaseCode=AE
  Math Function : Math  Operator=transpose  SaturateOnIntegerOverflow=on
  Matrix Multiply : Product  Multiplication=Matrix(*)
  Matrix Multiply1 : Product  Multiplication=Matrix(*)
  SRP Torque : MATLAB Function  TreatAsAtomicUnit=on
  Stop Simulation : Stop
  Sum : Sum  Inputs=5
  To Workspace : ToWorkspace  VariableName=tor_gg_earth  SampleTime=-1
  To Workspace1 : ToWorkspace  VariableName=tor_gg_moon  SampleTime=-1
  To Workspace2 : ToWorkspace  VariableName=tor_srp  SampleTime=-1
  To Workspace3 : ToWorkspace  VariableName=tor_tot_body  SampleTime=-1
  To Workspace4 : ToWorkspace  VariableName=f_SRP_body  SampleTime=-1
  "nT -> T" : Gain  Gain=10^-9
  Torques : Outport
  wires:
  r_eci/1 -> Matrix Multiply1/2, Grav gradient earth/1(r_eci)
  Sum/1 -> To Workspace3/1, Torques/1
  Grav gradient earth/1(Torque_body) -> To Workspace/1, Sum/1
  Grav gradient moon/1(Torque_body) -> To Workspace1/1, Sum/2
  Aero Torque/1(tor) -> Sum/3
  Force_aero_body/1 -> Aero Torque/1(f_aero_body)
  Force_SRP_body/1 -> Gain/1
  SRP Torque/1(tor) -> To Workspace2/1, Sum/4
  Mag Torque/1 -> Sum/5
  Mag/1 -> "nT -> T"/1
  Constant/1 -> Aero Torque/2(moment_arms), SRP Torque/2(moment_arms)
  Constant1/1 -> Mag Torque/1
  "nT -> T"/1 -> Mag Torque/2
  Coordinate Transforms/1 -> Bus Selector/1
  Bus Selector/1 -> Grav gradient earth/2(R_eci2body), Matrix Multiply/2  "<R_eci2body>"
  Bus Selector/2 -> Matrix Multiply1/1, Math Function/1  "<R_eci2mci>"
  Math Function/1 -> Matrix Multiply/1
  Matrix Multiply/1 -> Grav gradient moon/2(R_mci2body)
  Matrix Multiply1/1 -> MATLAB Function/1(r_mci), Grav gradient moon/1(r_mci)
  Gain/1 -> To Workspace4/1, SRP Torque/1(f_SRP_body)
  MATLAB Function/1(y) -> Stop Simulation/1
  Constant2/1 -> MATLAB Function/2(r_moon)

== system ADCS_r2017b/Satellite Simulator/Kinematics/Backup Rotation Kinematics ==
  torque_body : Inport
  Adams Bashforth Integration : Subsystem
  Adams Bashforth Integration1 : Subsystem
  Constant : Constant  Value=SC.initial_state.e
  Constant1 : Constant  Value=SC.initial_state.w
  Constant2 : Constant  Value=delta_t
  Constant3 : Constant  Value=SC.mass_properties.inertia
  Constant4 : Constant  Value=delta_t
  Delay : Delay  DelayLength=1  InitialConditionSource=Input port  InitialCondition=0
      settings: InputPortMap=u0,p4
  Delay1 : Delay  DelayLength=1  InitialConditionSource=Input port  InitialCondition=0
      settings: InputPortMap=u0,p4
  Euler Equations : MATLAB Function  TreatAsAtomicUnit=on
  calc_e_dot : MATLAB Function  TreatAsAtomicUnit=on
  euler_angles : Outport
  w_body_eci : Outport  Port=2
  wires:
  Constant/1 -> Delay/2, Adams Bashforth Integration/1(x_initial)
  Constant2/1 -> Adams Bashforth Integration/3(dt)
  Adams Bashforth Integration/1(x) -> euler_angles/1, Delay/1
  calc_e_dot/1(e_dot) -> Adams Bashforth Integration/2(x_dot)
  Delay/1 -> calc_e_dot/1(e)
  Constant1/1 -> Adams Bashforth Integration1/1(x_initial), Delay1/2
  Adams Bashforth Integration1/1(x) -> w_body_eci/1, Delay1/1
  torque_body/1 -> Euler Equations/2(tor)
  Euler Equations/1(w_dot) -> Adams Bashforth Integration1/2(x_dot)
  Constant3/1 -> Euler Equations/3(I)
  Delay1/1 -> calc_e_dot/2(w), Euler Equations/1(w)
  Constant4/1 -> Adams Bashforth Integration1/3(dt)

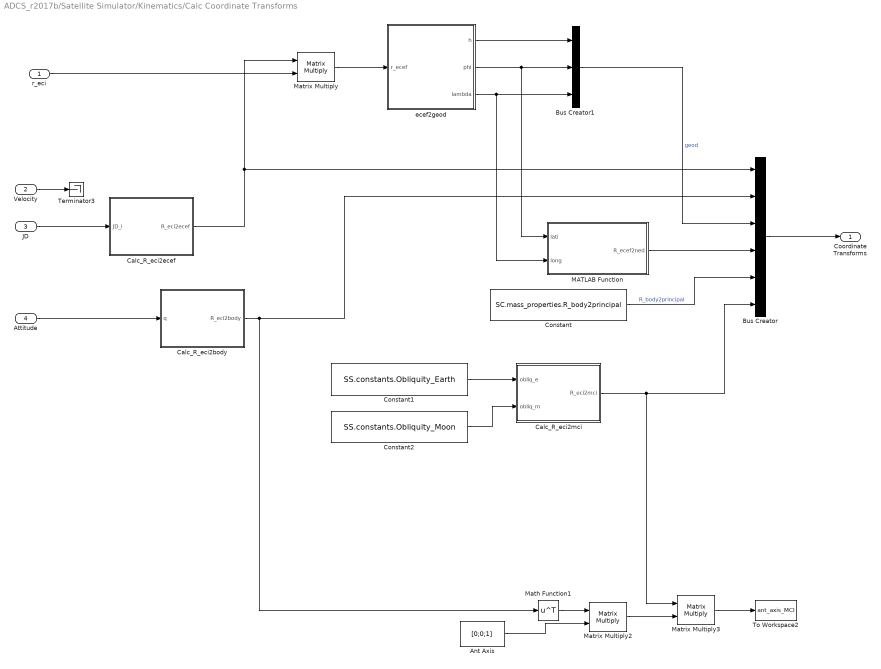
== system ADCS_r2017b/Satellite Simulator/Kinematics/Calc Coordinate Transforms ==
  r_eci : Inport  PortDimensions=3
  Velocity : Inport  Port=2
  JD : Inport  Port=3
  Attitude : Inport  Port=4
  Ant Axis : Constant  Value=[0;0;1]
  Bus Creator : BusCreator  Inputs=6
  Bus Creator1 : BusCreator  Inputs=3
  Calc_R_eci2body : MATLAB Function  TreatAsAtomicUnit=on
  Calc_R_eci2ecef : MATLAB Function  TreatAsAtomicUnit=on
  Calc_R_eci2mci : MATLAB Function  TreatAsAtomicUnit=on
  Constant : Constant  Value=SC.mass_properties.R_body2principal
  Constant1 : Constant  Value=SS.constants.Obliquity_Earth
  Constant2 : Constant  Value=SS.constants.Obliquity_Moon
  MATLAB Function : MATLAB Function  TreatAsAtomicUnit=on
  Math Function1 : Math  Operator=transpose  SaturateOnIntegerOverflow=on
  Matrix Multiply : Product  Multiplication=Matrix(*)
  Matrix Multiply2 : Product  Multiplication=Matrix(*)
  Matrix Multiply3 : Product  Multiplication=Matrix(*)
  Terminator3 : Terminator
  To Workspace2 : ToWorkspace  VariableName=ant_axis_MCI  SampleTime=-1
  ecef2geod : MATLAB Function  TreatAsAtomicUnit=on
  Coordinate Transforms : Outport
  wires:
  Bus Creator/1 -> Coordinate Transforms/1
  Attitude/1 -> Calc_R_eci2body/1(q)
  JD/1 -> Calc_R_eci2ecef/1(JD_i)
  r_eci/1 -> Matrix Multiply/2
  Matrix Multiply/1 -> ecef2geod/1(r_ecef)
  Calc_R_eci2ecef/1(R_eci2ecef) -> Matrix Multiply/1, Bus Creator/1
  ecef2geod/1(h) -> Bus Creator1/1
  ecef2geod/2(phi) -> MATLAB Function/1(lati), Bus Creator1/2
  ecef2geod/3(lambda) -> MATLAB Function/2(long), Bus Creator1/3
  Calc_R_eci2body/1(R_eci2body) -> Math Function1/1, Bus Creator/2
  Velocity/1 -> Terminator3/1
  Bus Creator1/1 -> Bus Creator/3  "geod"
  MATLAB Function/1(R_ecef2ned) -> Bus Creator/4
  Constant/1 -> Bus Creator/5  "R_body2principal"
  Calc_R_eci2mci/1(R_eci2mci) -> Matrix Multiply3/1, Bus Creator/6
  Constant1/1 -> Calc_R_eci2mci/1(obliq_e)
  Constant2/1 -> Calc_R_eci2mci/2(obliq_m)
  Math Function1/1 -> Matrix Multiply2/1
  Ant Axis/1 -> Matrix Multiply2/2
  Matrix Multiply2/1 -> Matrix Multiply3/2
  Matrix Multiply3/1 -> To Workspace2/1

== system ADCS_r2017b/Satellite Simulator/Kinematics/Position Kinematics ==
  a_eci : Inport
  Adams Bashforth Integration1 : Subsystem  TreatAsAtomicUnit=on
  Adams Bashforth Integration2 : Subsystem  TreatAsAtomicUnit=on
  Constant : Constant  Value=SC.initial_state.r_eci
  Constant1 : Constant  Value=SC.initial_state.v_eci
  Constant2 : Constant  Value=delta_t
  To Workspace : ToWorkspace  VariableName=r_eci  SampleTime=-1
  To Workspace1 : ToWorkspace  VariableName=v_eci  SampleTime=-1
  r_eci : Outport
  v_eci : Outport  Port=2
  wires:
  a_eci/1 -> Adams Bashforth Integration1/2(x_dot)
  Constant2/1 -> Adams Bashforth Integration2/3(dt), Adams Bashforth Integration1/3(dt)
  Constant/1 -> Adams Bashforth Integration2/1(x_initial)
  Constant1/1 -> Adams Bashforth Integration1/1(x_initial)
  Adams Bashforth Integration1/1(x) -> Adams Bashforth Integration2/2(x_dot), To Workspace1/1, v_eci/1
  Adams Bashforth Integration2/1(x) -> r_eci/1, To Workspace/1

== system ADCS_r2017b/Satellite Simulator/Kinematics/Rotation Kinematics ==
  torque_body : Inport
  Adams Bashforth Integration : Subsystem  TreatAsAtomicUnit=on
  Adams Bashforth Integration1 : Subsystem  TreatAsAtomicUnit=on
  Constant : Constant  Value=SC.initial_state.q
  Constant1 : Constant  Value=SC.initial_state.w
  Constant2 : Constant  Value=delta_t
  Constant3 : Constant  Value=SC.mass_properties.inertia
  Constant4 : Constant  Value=delta_t
  Delay : Delay  DelayLength=1  InitialConditionSource=Input port  InitialCondition=0
      settings: InputPortMap=u0,p4
  Delay1 : Delay  DelayLength=1  InitialConditionSource=Input port  InitialCondition=0
      settings: InputPortMap=u0,p4
  Euler Equations : MATLAB Function  TreatAsAtomicUnit=on
  calc_q_dot : MATLAB Function  TreatAsAtomicUnit=on
  q : Outport
  w_body_eci : Outport  Port=2
  wires:
  Constant/1 -> Delay/2, Adams Bashforth Integration/1(x_initial)
  Constant2/1 -> Adams Bashforth Integration/3(dt)
  calc_q_dot/1(q_dot) -> Adams Bashforth Integration/2(x_dot)
  Delay/1 -> calc_q_dot/1(q)
  Constant1/1 -> Adams Bashforth Integration1/1(x_initial), Delay1/2
  Adams Bashforth Integration1/1(x) -> w_body_eci/1, Delay1/1
  torque_body/1 -> Euler Equations/2(tor)
  Euler Equations/1(w_dot) -> Adams Bashforth Integration1/2(x_dot)
  Constant3/1 -> Euler Equations/3(I)
  Delay1/1 -> calc_q_dot/2(w), Euler Equations/1(w)
  Constant4/1 -> Adams Bashforth Integration1/3(dt)
  Adams Bashforth Integration/1(x) -> q/1, Delay/1

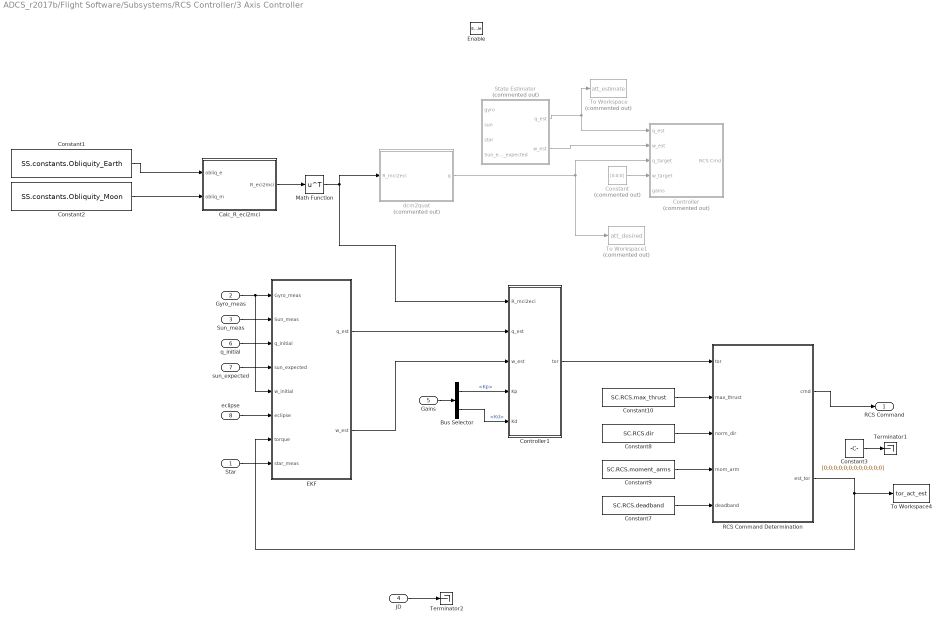
== system ADCS_r2017b/Flight Software/Subsystems/RCS Controller/3 Axis Controller ==
  Star : Inport
  Gyro_meas : Inport  Port=2
  Sun_meas : Inport  Port=3
  JD : Inport  Port=4
  Gains : Inport  Port=5
  q_initial : Inport  Port=6
  sun_expected : Inport  Port=7
  eclipse : Inport  Port=8
  Enable : EnablePort
  Bus Selector : BusSelector  OutputSignals=Kp,Kd
  Calc_R_eci2mci : MATLAB Function  TreatAsAtomicUnit=on
  Constant : Constant  Commented=on  Value=[0;0;0]
  Constant1 : Constant  Value=SS.constants.Obliquity_Earth
  Constant10 : Constant  Value=SC.RCS.max_thrust
  Constant2 : Constant  Value=SS.constants.Obliquity_Moon
  Constant3 : Constant  Value=[0;0;0;0;0;0;0;0;0;0;0;0]
  Constant7 : Constant  Value=SC.RCS.deadband
  Constant8 : Constant  Value=SC.RCS.dir
  Constant9 : Constant  Value=SC.RCS.moment_arms
  Controller : Subsystem  Commented=on
  Controller1 : MATLAB Function  TreatAsAtomicUnit=on
  EKF : Subsystem
  Math Function : Math  Operator=transpose  SaturateOnIntegerOverflow=on
  RCS Command Determination : MATLAB Function  TreatAsAtomicUnit=on
  State Estimator : Subsystem  Commented=on
  Terminator1 : Terminator
  Terminator2 : Terminator
  To Workspace : ToWorkspace  Commented=on  VariableName=att_estimate  SampleTime=-1
  To Workspace1 : ToWorkspace  Commented=on  VariableName=att_desired  SampleTime=-1
  To Workspace4 : ToWorkspace  VariableName=tor_act_est  SampleTime=-1
  dcm2quat : MATLAB Function  Commented=on  TreatAsAtomicUnit=on
  RCS Command : Outport
  wires:
  State Estimator/1(q_est) -> To Workspace/1, Controller/1(q_est)
  State Estimator/2(w_est) -> Controller/2(w_est)
  Constant/1 -> Controller/4(w_target)
  Constant1/1 -> Calc_R_eci2mci/1(obliq_e)
  Constant2/1 -> Calc_R_eci2mci/2(obliq_m)
  dcm2quat/1(q) -> Controller/3(q_target), To Workspace1/1
  Calc_R_eci2mci/1(R_eci2mci) -> Math Function/1
  Math Function/1 -> Controller1/1(R_mci2eci), dcm2quat/1(R_mci2eci)
  q_initial/1 -> EKF/3(q_initial)
  eclipse/1 -> EKF/6(eclipse)
  Sun_meas/1 -> EKF/2(Sun_meas)
  RCS Command Determination/1(cmd) -> RCS Command/1
  EKF/2(w_est) -> Controller1/3(w_est)
  EKF/1(q_est) -> Controller1/2(q_est)
  Bus Selector/2 -> Controller1/5(Kd)  "<Kd>"
  Gains/1 -> Bus Selector/1
  Controller1/1(tor) -> RCS Command Determination/1(tor)
  Constant3/1 -> Terminator1/1
  Constant8/1 -> RCS Command Determination/3(norm_dir)
  JD/1 -> Terminator2/1
  Gyro_meas/1 -> EKF/5(w_initial), EKF/1(Gyro_meas)
  Bus Selector/1 -> Controller1/4(Kp)  "<Kp>"
  Constant10/1 -> RCS Command Determination/2(max_thrust)
  Constant9/1 -> RCS Command Determination/4(mom_arm)
  Constant7/1 -> RCS Command Determination/5(deadband)
  sun_expected/1 -> EKF/4(sun_expected)
  Star/1 -> EKF/8(star_meas)
  RCS Command Determination/2(est_tor) -> To Workspace4/1, EKF/7(torque)

== system ADCS_r2017b/Flight Software/Subsystems/RCS Controller/Environment ==
  JD : Inport
  Constant2 : Constant  Value=SS.constants.orbit_coef.mop_moon_eph_coeff
  Constant3 : Constant  Value=SS.constants.orbit_coef.mop_moon_jd_lookup
  Constant4 : Constant  Value=SS.constants.orbit_coef.sol_emb_eph_coeff
  Constant5 : Constant  Value=SS.constants.orbit_coef.sol_sun_eph_coeff
  Constant6 : Constant  Value=SS.constants.orbit_coef.sol_sun_jd_lookup
  Moon position in ECI : MATLAB Function  TreatAsAtomicUnit=on
  Sun position in ECI : MATLAB Function  TreatAsAtomicUnit=on
  sun_eci : Outport
  moon_eci : Outport  Port=2
  wires:
  Constant4/1 -> Sun position in ECI/3(sol_emb_eph_coeff)
  Moon position in ECI/1(moon_eci) -> moon_eci/1, Sun position in ECI/2(moon_eci)
  Constant5/1 -> Sun position in ECI/4(sol_sun_eph_coeff)
  Constant3/1 -> Moon position in ECI/3(mop_moon_jd_lookup)
  Constant2/1 -> Moon position in ECI/2(mop_moon_eph_coeff)
  Constant6/1 -> Sun position in ECI/5(sol_sun_jd_lookup)
  JD/1 -> Moon position in ECI/1(JD_tt), Sun position in ECI/1(JD_tt)
  Sun position in ECI/1(sun_eci) -> sun_eci/1

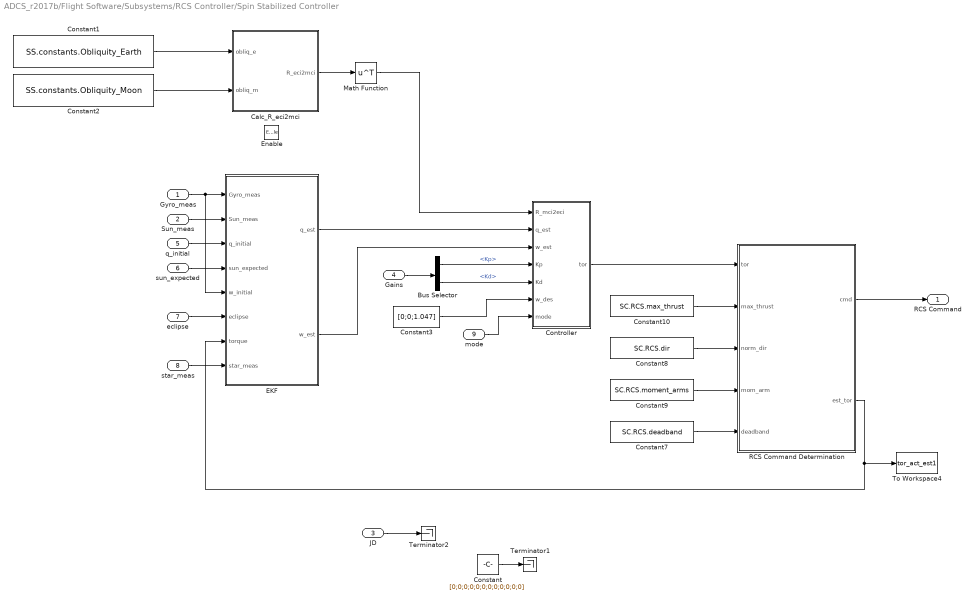
== system ADCS_r2017b/Flight Software/Subsystems/RCS Controller/Spin Stabilized Controller ==
  Gyro_meas : Inport
  Sun_meas : Inport  Port=2
  JD : Inport  Port=3
  Gains : Inport  Port=4
  q_initial : Inport  Port=5
  sun_expected : Inport  Port=6
  eclipse : Inport  Port=7
  star_meas : Inport  Port=8
  mode : Inport  Port=9
  Enable : EnablePort
  Bus Selector : BusSelector  OutputSignals=Kp,Kd
  Calc_R_eci2mci : MATLAB Function  TreatAsAtomicUnit=on
  Constant : Constant  Value=[0;0;0;0;0;0;0;0;0;0;0;0]
  Constant1 : Constant  Value=SS.constants.Obliquity_Earth
  Constant10 : Constant  Value=SC.RCS.max_thrust
  Constant2 : Constant  Value=SS.constants.Obliquity_Moon
  Constant3 : Constant  Value=[0;0;1.047]
  Constant7 : Constant  Value=SC.RCS.deadband
  Constant8 : Constant  Value=SC.RCS.dir
  Constant9 : Constant  Value=SC.RCS.moment_arms
  Controller : MATLAB Function  TreatAsAtomicUnit=on
  EKF : Subsystem
  Math Function : Math  Operator=transpose  SaturateOnIntegerOverflow=on
  RCS Command Determination : MATLAB Function  TreatAsAtomicUnit=on
  Terminator1 : Terminator
  Terminator2 : Terminator
  To Workspace4 : ToWorkspace  VariableName=tor_act_est1  SampleTime=-1
  RCS Command : Outport
  wires:
  Gains/1 -> Bus Selector/1
  JD/1 -> Terminator2/1
  Constant/1 -> Terminator1/1
  RCS Command Determination/1(cmd) -> RCS Command/1
  Constant7/1 -> RCS Command Determination/5(deadband)
  Constant8/1 -> RCS Command Determination/3(norm_dir)
  Constant9/1 -> RCS Command Determination/4(mom_arm)
  Constant10/1 -> RCS Command Determination/2(max_thrust)
  Gyro_meas/1 -> EKF/5(w_initial), EKF/1(Gyro_meas)
  Sun_meas/1 -> EKF/2(Sun_meas)
  eclipse/1 -> EKF/6(eclipse)
  sun_expected/1 -> EKF/4(sun_expected)
  q_initial/1 -> EKF/3(q_initial)
  EKF/1(q_est) -> Controller/2(q_est)
  EKF/2(w_est) -> Controller/3(w_est)
  Controller/1(tor) -> RCS Command Determination/1(tor)
  Bus Selector/1 -> Controller/4(Kp)  "<Kp>"
  Bus Selector/2 -> Controller/5(Kd)  "<Kd>"
  RCS Command Determination/2(est_tor) -> To Workspace4/1, EKF/7(torque)
  Calc_R_eci2mci/1(R_eci2mci) -> Math Function/1
  Constant1/1 -> Calc_R_eci2mci/1(obliq_e)
  Constant2/1 -> Calc_R_eci2mci/2(obliq_m)
  Math Function/1 -> Controller/1(R_mci2eci)
  Constant3/1 -> Controller/6(w_des)
  star_meas/1 -> EKF/8(star_meas)
  mode/1 -> Controller/7(mode)

== system ADCS_r2017b/Flight Software/Subsystems/RCS Controller/Spin Up Controller ==
  Gyro : Inport
  Sun : Inport  Port=2
  Time : Inport  Port=3
  Gains : Inport  Port=4
  Enable : EnablePort
  Constant : Constant  Value=[0;0;0;0;0;0;0;0;0;0;0;0]
  Terminator{,2..4} (4 alike) : Terminator
  RCS Command : Outport
  wires:
  Gains/1 -> Terminator3/1
  Gyro/1 -> Terminator4/1
  Time/1 -> Terminator2/1
  Constant/1 -> RCS Command/1
  Sun/1 -> Terminator/1

== system ADCS_r2017b/Flight Software/Subsystems/Sensor Processing/Discrete Low Pass Filter ==
  Raw : Inport
  w_cutoff : Inport  Port=2
  dt : Inport  Port=3
  Constant1 : Constant
  Delay : Delay  DelayLength=1  InitialCondition=0
  Divide : Product  Inputs=**
  Exp : Math  SaturateOnIntegerOverflow=on
  Gain : Gain  Gain=-1
  Product : Product
  Product1 : Product
  Sum : Sum  Inputs=|++
  Sum2 : Sum  Inputs=+-
  Filtered : Outport
  wires:
  w_cutoff/1 -> Divide/1
  dt/1 -> Divide/2
  Divide/1 -> Gain/1
  Raw/1 -> Product/1
  Product/1 -> Sum/1
  Sum/1 -> Delay/1, Filtered/1
  Product1/1 -> Sum/2
  Gain/1 -> Exp/1
  Exp/1 -> Product1/1, Sum2/2  "Alpha"
  Constant1/1 -> Sum2/1
  Sum2/1 -> Product/2
  Delay/1 -> Product1/2

== system ADCS_r2017b/Flight Software/Subsystems/Sensor Processing/Discrete Low Pass Filter1 ==
  Raw : Inport
  w_cutoff : Inport  Port=2
  dt : Inport  Port=3
  Constant1 : Constant
  Delay : Delay  DelayLength=1  InitialCondition=0
  Divide : Product  Inputs=**
  Exp : Math  SaturateOnIntegerOverflow=on
  Gain : Gain  Gain=-1
  Product : Product
  Product1 : Product
  Sum : Sum  Inputs=|++
  Sum2 : Sum  Inputs=+-
  Filtered : Outport
  wires:
  w_cutoff/1 -> Divide/1
  dt/1 -> Divide/2
  Divide/1 -> Gain/1
  Raw/1 -> Product/1
  Product/1 -> Sum/1
  Sum/1 -> Delay/1, Filtered/1
  Product1/1 -> Sum/2
  Gain/1 -> Exp/1
  Exp/1 -> Product1/1, Sum2/2  "Alpha"
  Constant1/1 -> Sum2/1
  Sum2/1 -> Product/2
  Delay/1 -> Product1/2

== system ADCS_r2017b/Flight Software/Subsystems/Sensor Processing/Discrete Low Pass Filter2 ==
  Raw : Inport
  w_cutoff : Inport  Port=2
  dt : Inport  Port=3
  Constant1 : Constant
  Delay : Delay  DelayLength=1  InitialCondition=0
  Divide : Product  Inputs=**
  Exp : Math  SaturateOnIntegerOverflow=on
  Gain : Gain  Gain=-1
  Product : Product
  Product1 : Product
  Sum : Sum  Inputs=|++
  Sum2 : Sum  Inputs=+-
  Filtered : Outport
  wires:
  w_cutoff/1 -> Divide/1
  dt/1 -> Divide/2
  Divide/1 -> Gain/1
  Raw/1 -> Product/1
  Product/1 -> Sum/1
  Sum/1 -> Delay/1, Filtered/1
  Product1/1 -> Sum/2
  Gain/1 -> Exp/1
  Exp/1 -> Product1/1, Sum2/2  "Alpha"
  Constant1/1 -> Sum2/1
  Sum2/1 -> Product/2
  Delay/1 -> Product1/2

== system ADCS_r2017b/Flight Software/Subsystems/Sensor Processing/Discrete Low Pass Filter3 ==
  Raw : Inport
  w_cutoff : Inport  Port=2
  dt : Inport  Port=3
  Constant1 : Constant
  Delay : Delay  DelayLength=1  InitialCondition=0
  Divide : Product  Inputs=**
  Exp : Math  SaturateOnIntegerOverflow=on
  Gain : Gain  Gain=-1
  Product : Product
  Product1 : Product
  Sum : Sum  Inputs=|++
  Sum2 : Sum  Inputs=+-
  Filtered : Outport
  wires:
  w_cutoff/1 -> Divide/1
  dt/1 -> Divide/2
  Divide/1 -> Gain/1
  Raw/1 -> Product/1
  Product/1 -> Sum/1
  Sum/1 -> Delay/1, Filtered/1
  Product1/1 -> Sum/2
  Gain/1 -> Exp/1
  Exp/1 -> Product1/1, Sum2/2  "Alpha"
  Constant1/1 -> Sum2/1
  Sum2/1 -> Product/2
  Delay/1 -> Product1/2

== system ADCS_r2017b/Satellite Simulator/External Forces and Torques/External Torques/Grav gradient earth ==
  r_eci : Inport
  R_eci2body : Inport  Port=2
  3x3 Cross Product : sharedutil/3x3 Cross Product
      settings: SourceProductBaseCode=AE
  Constant : Constant  Value=SC.mass_properties.inertia
  Constant1 : Constant  Value=SS.constants.GM_Earth
  MATLAB Function : MATLAB Function  TreatAsAtomicUnit=on
  Matrix Multiply : Product  Multiplication=Matrix(*)
  Matrix Multiply1 : Product  Multiplication=Matrix(*)
  Normalize Vector : vrlib/Utilities/Normalize Vector  maxzero=0
      settings: SourceProductName=Simulink 3D Animation  SourceProductBaseCode=VR
  Torque_body : Outport
  wires:
  R_eci2body/1 -> Matrix Multiply/1
  r_eci/1 -> MATLAB Function/2(r_eci), Matrix Multiply/2
  Matrix Multiply/1 -> Normalize Vector/1
  Constant/1 -> Matrix Multiply1/1
  Normalize Vector/1 -> 3x3 Cross Product/1, Matrix Multiply1/2
  Matrix Multiply1/1 -> 3x3 Cross Product/2
  3x3 Cross Product/1 -> MATLAB Function/1(rIr)
  Constant1/1 -> MATLAB Function/3(GM)
  MATLAB Function/1(tor) -> Torque_body/1

== system ADCS_r2017b/Satellite Simulator/External Forces and Torques/External Torques/Grav gradient moon ==
  r_mci : Inport
  R_mci2body : Inport  Port=2
  3x3 Cross Product : sharedutil/3x3 Cross Product
      settings: SourceProductBaseCode=AE
  Constant : Constant  Value=SC.mass_properties.inertia
  Constant1 : Constant  Value=SS.constants.GM_Moon
  MATLAB Function : MATLAB Function  TreatAsAtomicUnit=on
  Matrix Multiply : Product  Multiplication=Matrix(*)
  Matrix Multiply1 : Product  Multiplication=Matrix(*)
  Normalize Vector : vrlib/Utilities/Normalize Vector  maxzero=0
      settings: SourceProductName=Simulink 3D Animation  SourceProductBaseCode=VR
  Torque_body : Outport
  wires:
  R_mci2body/1 -> Matrix Multiply/1
  r_mci/1 -> MATLAB Function/2(r_mci), Matrix Multiply/2
  Matrix Multiply/1 -> Normalize Vector/1
  Constant/1 -> Matrix Multiply1/1
  Normalize Vector/1 -> 3x3 Cross Product/1, Matrix Multiply1/2
  Matrix Multiply1/1 -> 3x3 Cross Product/2
  3x3 Cross Product/1 -> MATLAB Function/1(rIr)
  Constant1/1 -> MATLAB Function/3(GM)
  MATLAB Function/1(tor) -> Torque_body/1

== system ADCS_r2017b/Satellite Simulator/Kinematics/Backup Rotation Kinematics/Adams Bashforth Integration ==
  x_initial : Inport
  x_dot : Inport  Port=2
  dt : Inport  Port=3
  Delay : Delay  DelayLength=1  InitialConditionSource=Input port  InitialCondition=0
      settings: InputPortMap=u0,p4
  Delay1 : Delay  DelayLength=1  InitialConditionSource=Input port  InitialCondition=0
      settings: InputPortMap=u0,p4
  Delay2 : Delay  DelayLength=1  InitialConditionSource=Input port  InitialCondition=0
      settings: InputPortMap=u0,p4
  Gain : Gain  Gain=23/12
  Gain1 : Gain  Gain=-16/12
  Gain2 : Gain  Gain=5/12
  Product : Product
  Sum : Sum  Inputs=|++
  Sum1 : Sum  Inputs=+++
  x : Outport
  wires:
  x_initial/1 -> Delay/2
  Delay/1 -> Sum/1
  Sum/1 -> Delay/1, x/1
  Delay1/1 -> Delay2/1, Gain1/1
  x_dot/1 -> Delay2/2, Delay1/2, Delay1/1, Gain/1
  Gain1/1 -> Sum1/2
  Gain/1 -> Sum1/1
  Gain2/1 -> Sum1/3
  Sum1/1 -> Product/1
  dt/1 -> Product/2
  Product/1 -> Sum/2
  Delay2/1 -> Gain2/1

== system ADCS_r2017b/Satellite Simulator/Kinematics/Backup Rotation Kinematics/Adams Bashforth Integration1 ==
  x_initial : Inport
  x_dot : Inport  Port=2
  dt : Inport  Port=3
  Delay : Delay  DelayLength=1  InitialConditionSource=Input port  InitialCondition=0
      settings: InputPortMap=u0,p4
  Delay1 : Delay  DelayLength=1  InitialConditionSource=Input port  InitialCondition=0
      settings: InputPortMap=u0,p4
  Delay2 : Delay  DelayLength=1  InitialConditionSource=Input port  InitialCondition=0
      settings: InputPortMap=u0,p4
  Gain : Gain  Gain=23/12
  Gain1 : Gain  Gain=-16/12
  Gain2 : Gain  Gain=5/12
  Product : Product
  Sum : Sum  Inputs=|++
  Sum1 : Sum  Inputs=+++
  x : Outport
  wires:
  x_initial/1 -> Delay/2
  Delay/1 -> Sum/1
  Sum/1 -> Delay/1, x/1
  Delay1/1 -> Delay2/1, Gain1/1
  x_dot/1 -> Delay2/2, Delay1/2, Delay1/1, Gain/1
  Gain1/1 -> Sum1/2
  Gain/1 -> Sum1/1
  Gain2/1 -> Sum1/3
  Sum1/1 -> Product/1
  dt/1 -> Product/2
  Product/1 -> Sum/2
  Delay2/1 -> Gain2/1

== system ADCS_r2017b/Satellite Simulator/Kinematics/Position Kinematics/Adams Bashforth Integration1 ==
  x_initial : Inport
  x_dot : Inport  Port=2
  dt : Inport  Port=3
  Delay : Delay  DelayLength=1  InitialConditionSource=Input port  InitialCondition=0
      settings: InputPortMap=u0,p4
  Delay1 : Delay  DelayLength=1  InitialConditionSource=Input port  InitialCondition=0
      settings: InputPortMap=u0,p4
  Delay2 : Delay  DelayLength=1  InitialConditionSource=Input port  InitialCondition=0
      settings: InputPortMap=u0,p4
  Gain : Gain  Gain=23/12
  Gain1 : Gain  Gain=-16/12
  Gain2 : Gain  Gain=5/12
  Product : Product
  Sum : Sum  Inputs=|++
  Sum1 : Sum  Inputs=+++
  x : Outport
  wires:
  x_initial/1 -> Delay/2
  Delay/1 -> Sum/1
  Sum/1 -> Delay/1, x/1
  Delay1/1 -> Delay2/1, Gain1/1
  x_dot/1 -> Delay2/2, Delay1/2, Delay1/1, Gain/1
  Gain1/1 -> Sum1/2
  Gain/1 -> Sum1/1
  Gain2/1 -> Sum1/3
  Sum1/1 -> Product/1
  dt/1 -> Product/2
  Product/1 -> Sum/2
  Delay2/1 -> Gain2/1
